simulink model "SpacecraftPowerManagement"  (R2023b)
settings: Solver=ode45  StartTime=0.0  StopTime=10800  RelTol=1e-6
settings Model: Creator=USER  LastModifiedBy=USER

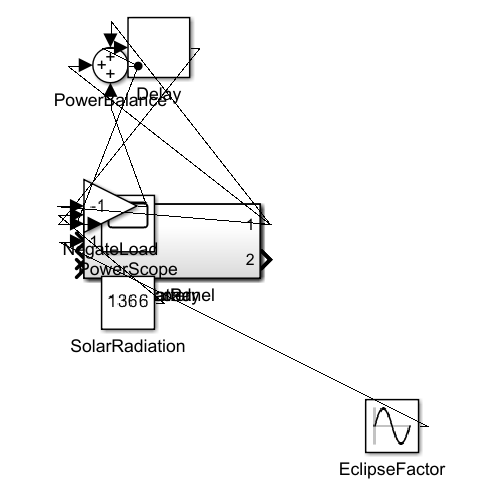
[thumbnail: Simulink's stored preview of the top-level diagram]
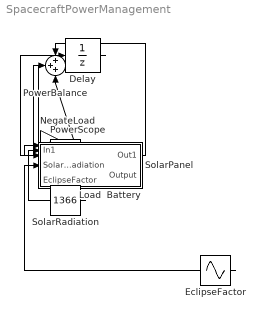
== system SpacecraftPowerManagement ==
  Battery : Subsystem
  Delay : UnitDelay  SampleTime=0.01  HasFrameUpgradeWarning=on
  EclipseFactor : Sin  Amplitude=0.5  Bias=0.5  Frequency=1/5400  SampleTime=0
  Load : Subsystem
  NegateLoad : Gain  Gain=-1
  PowerBalance : Sum  Inputs=+++
  PowerScope : Scope
  SolarPanel : Subsystem
  SolarRadiation : Constant  Value=1366
  wires:
  SolarRadiation/1 -> SolarPanel/1(In1)
  EclipseFactor/1 -> SolarPanel/2(SolarRadiation)
  SolarPanel/1(Out1) -> PowerBalance/1
  Battery/1(Out1) -> PowerBalance/2
  Load/1(Out1) -> NegateLoad/1
  NegateLoad/1 -> PowerBalance/3
  PowerBalance/1 -> Delay/1, PowerScope/1
  Delay/1 -> Battery/1(In1)

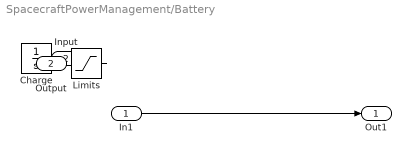
== system SpacecraftPowerManagement/Battery ==
  In1 : Inport
  Input : Inport  Port=2
  Charge : Integrator  InitialCondition=1000
  Limits : Saturate  UpperLimit=2000  LowerLimit=0
  Out1 : Outport
  Output : Outport  Port=2
  wires:
  In1/1 -> Out1/1
  Input/1 -> Charge/1
  Charge/1 -> Limits/1
  Limits/1 -> Output/1

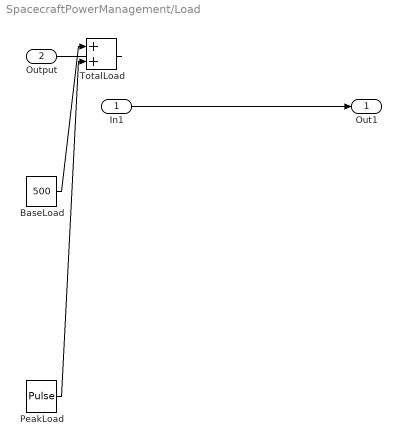
== system SpacecraftPowerManagement/Load ==
  In1 : Inport
  BaseLoad : Constant  Value=500
  PeakLoad : DiscretePulseGenerator  PulseType=Time based  Amplitude=1000  Period=3600  PulseWidth=10
  TotalLoad : Sum
  Out1 : Outport
  Output : Outport  Port=2
  wires:
  In1/1 -> Out1/1
  BaseLoad/1 -> TotalLoad/1
  PeakLoad/1 -> TotalLoad/2
  TotalLoad/1 -> Output/1

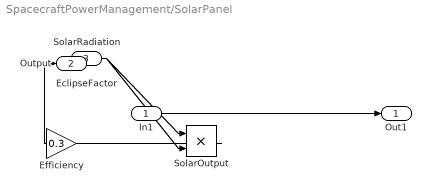
== system SpacecraftPowerManagement/SolarPanel ==
  In1 : Inport
  SolarRadiation : Inport  Port=2
  EclipseFactor : Inport  Port=3
  Efficiency : Gain  Gain=0.3
  SolarOutput : Product
  Out1 : Outport
  Output : Outport  Port=2
  wires:
  In1/1 -> Out1/1
  SolarRadiation/1 -> SolarOutput/1
  EclipseFactor/1 -> SolarOutput/2
  SolarOutput/1 -> Efficiency/1
  Efficiency/1 -> Output/1
